simulink subsystem "Motor_Model_Simulink"  (R2022b)
settings: Solver=VariableStepAuto  StartTime=0.0  StopTime=10.0  RelTol=1e-3
undefined symbols (not defined in the file or in its folder): bridge, motor
settings Model: Creator=gotta  LastModifiedBy=gotta

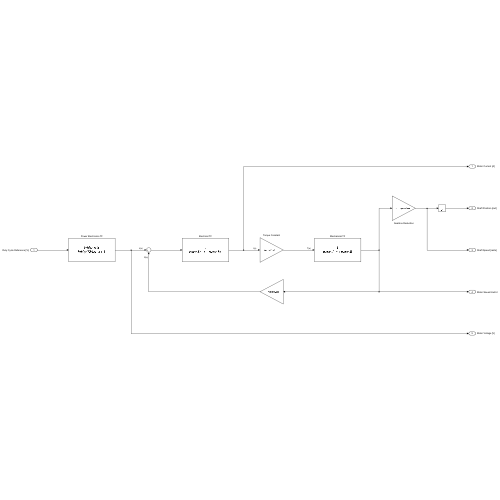
[thumbnail: Simulink's stored preview of the top-level diagram]
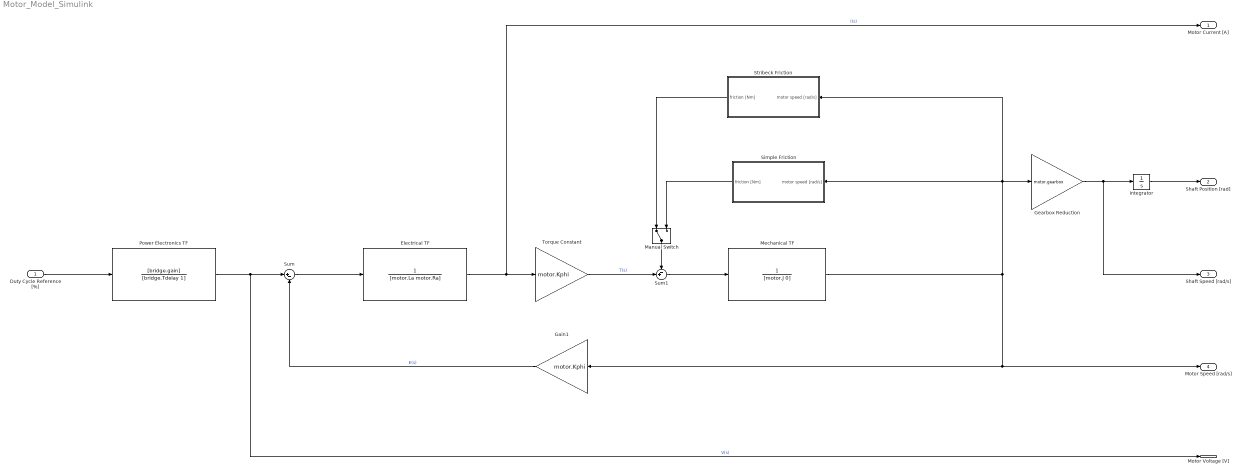
== system Motor_Model_Simulink ==
  Duty Cycle Reference [%] : Inport
  Electrical TF : TransferFcn  Denominator=[motor.La motor.Ra]
  Gain1 : Gain  Gain=motor.Kphi
  Gearbox Reduction : Gain  Gain=motor.gearbox
  Integrator : Integrator
  Manual Switch : ManualSwitch
  Mechanical TF : TransferFcn  Denominator=[motor.J 0]
  Power Electronics TF : TransferFcn  Numerator=[bridge.gain]  Denominator=[bridge.Tdelay 1]
  Simple Friction : Subsystem
  Stribeck Friction : Subsystem
  Sum : Sum  Inputs=|+-
  Sum1 : Sum  Inputs=-+|
  Torque Constant : Gain  Gain=motor.Kphi
  Motor Current [A] : Outport
  Shaft Position [rad] : Outport  Port=2
  Shaft Speed [rad/s] : Outport  Port=3
  Motor Speed [rad/s] : Outport  Port=4
  Motor Voltage [V] : Outport  Port=5
  wires:
  Mechanical TF/1 -> Gearbox Reduction/1, Stribeck Friction/1(motor speed [rad/s]), Simple Friction/1(motor speed [rad/s]), Motor Speed [rad/s]/1, Gain1/1
  Sum/1 -> Electrical TF/1
  Power Electronics TF/1 -> Motor Voltage [V]/1, Sum/1  "V(s)"
  Torque Constant/1 -> Sum1/2  "T(s)"
  Sum1/1 -> Mechanical TF/1
  Gearbox Reduction/1 -> Integrator/1, Shaft Speed [rad/s]/1
  Integrator/1 -> Shaft Position [rad]/1
  Duty Cycle Reference [%]/1 -> Power Electronics TF/1
  Electrical TF/1 -> Torque Constant/1, Motor Current [A]/1  "I(s)"
  Gain1/1 -> Sum/2  "E(s)"
  Manual Switch/1 -> Sum1/1
  Simple Friction/1(friction [Nm]) -> Manual Switch/2
  Stribeck Friction/1(friction [Nm]) -> Manual Switch/1

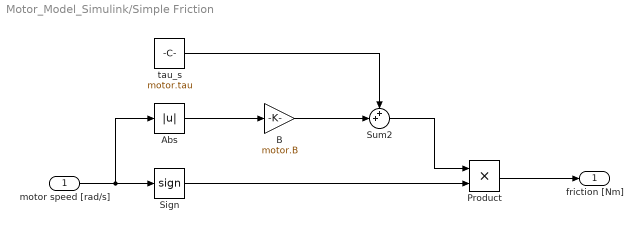
== system Motor_Model_Simulink/Simple Friction ==
  motor speed [rad/s] : Inport
  Abs : Abs  SaturateOnIntegerOverflow=off
  B : Gain  Gain=motor.B
  Product : Product
  Sign : Signum
  Sum2 : Sum  Inputs=++|
  tau_s : Constant  Value=motor.tau
  friction [Nm] : Outport
  wires:
  motor speed [rad/s]/1 -> Abs/1, Sign/1
  Sign/1 -> Product/2
  Product/1 -> friction [Nm]/1
  Abs/1 -> B/1
  tau_s/1 -> Sum2/1
  B/1 -> Sum2/2
  Sum2/1 -> Product/1

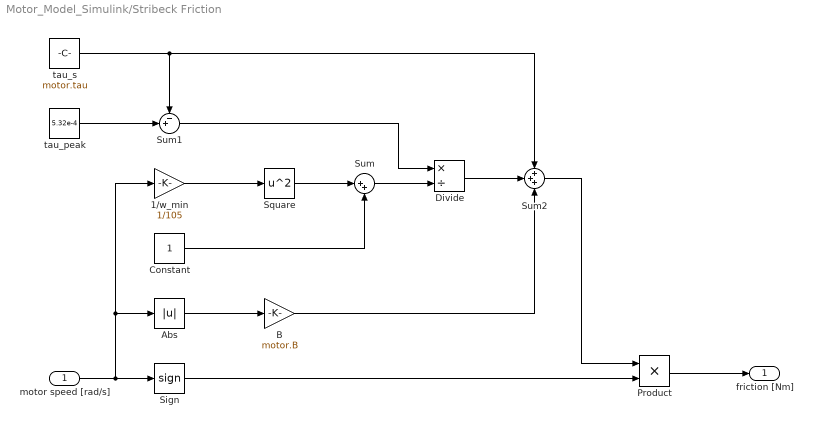
== system Motor_Model_Simulink/Stribeck Friction ==
  motor speed [rad/s] : Inport
  1/w_min : Gain  Gain=1/105
  Abs : Abs  SaturateOnIntegerOverflow=off
  B : Gain  Gain=motor.B
  Constant : Constant
  Divide : Product  Inputs=*/
  Product : Product
  Sign : Signum
  Square : Math  Operator=square
  Sum : Sum  Inputs=|++
  Sum1 : Sum  Inputs=-+|
  Sum2 : Sum  Inputs=+++
  tau_peak : Constant  Value=5.32e-4
  tau_s : Constant  Value=motor.tau
  friction [Nm] : Outport
  wires:
  Sum2/1 -> Product/1
  B/1 -> Sum2/3
  Divide/1 -> Sum2/2
  Sum1/1 -> Divide/1
  tau_s/1 -> Sum1/1, Sum2/1
  tau_peak/1 -> Sum1/2
  Sum/1 -> Divide/2
  Constant/1 -> Sum/2
  Square/1 -> Sum/1
  1/w_min/1 -> Square/1
  Abs/1 -> B/1
  Product/1 -> friction [Nm]/1
  Sign/1 -> Product/2
  motor speed [rad/s]/1 -> Sign/1, Abs/1, 1/w_min/1
